simulink model "nonlinearized"  (R2020a)
settings: Solver=ode45  StartTime=0.0  StopTime=1000  FixedStep=0.01  MaxStep=0.05  RelTol=1e-3
undefined symbols (not defined in the file): auniversal, CLRolla20breakpoint1, CLRolla20breakpoint2, CLRolla20data, CLRollbreakpoint1, CLRollbreakpoint2, CLRolldata, CLRollPdata, CLRollr30breakpoint1, CLRollr30breakpoint2, CLRollr30data, CLRollRdata, CMbreakpoint1, CMbreakpoint2, CMdata, CMQdata, CNa20breakpoint1, CNa20breakpoint2, CNa20data, CNbreakpoint1, CNbreakpoint2, CNdata, CNPdata, CNr30breakpoint1, CNr30breakpoint2, CNr30data, CNRdata, CXbreakpoint1, CXbreakpoint2, CXdata, CXQdata, CYPdata, CYRdata, CZbreakpoint, CZdata, CZQdata, Tidlebreakpoint1, Tidlebreakpoint2, Tidledata, Tmaxbreakpoint1, Tmaxbreakpoint2, Tmaxdata, Tmilbreakpoint1, Tmilbreakpoint2, Tmildata, y
libraries: aerolibatmos2 x1
settings Model: Creator=WIN10  LastModifiedBy=WangLindong
settings DataIOCC: ReturnWorkspaceOutputs=off
settings DebuggingCC: InitInArrayFormatMsg=none  ArithmeticOperatorsInVariantConditions=warning
settings SFSimCC: SimUseLocalCustomCode=off  CustomCodeUndefinedFunction=UseInterfaceOnly
settings RTWCC: RTWUseLocalCustomCode=off
settings CodeAppCC: StateflowObjectComments=on
settings SimscapeCC: SimscapeNormalizeSystem=off

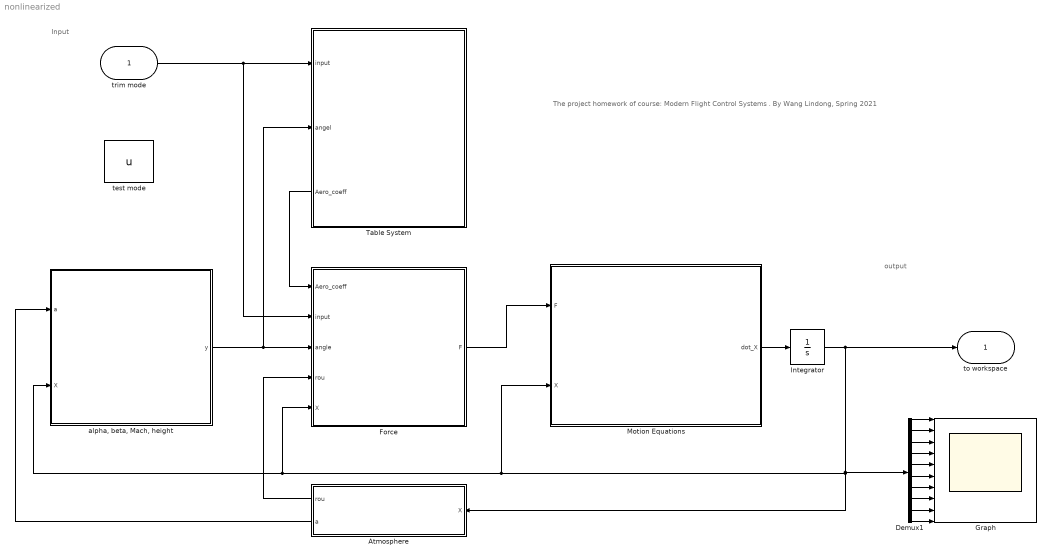
== system nonlinearized ==
  note: output
  note: Input
  note: The project homework of course: Modern Flight Control Systems . By Wang Lindong, Spring 2021
  trim mode : Inport
  Atmosphere : Subsystem
  Demux1 : Demux  Outputs=10
  Force : MATLAB Function  TreatAsAtomicUnit=on
  Graph : Scope  NumInputPorts=10
  Integrator : Integrator  InitialCondition=y
  Motion Equations : MATLAB Function  TreatAsAtomicUnit=on
  Table System : Subsystem
      settings: PortSchema="{\"entries\":[{\"content\":{\"sides\":[{\"content\":{\"connectorIds\":[\"In1\",\"In2\",\"Out1\"]},\"type\":\"ConnectorPlacement.EquallySpacedRectSide\",\"uuid\":\"a5097b1f-d505-459f-b2e6-571d27cac04d\"},{\"content\":{\"connectorIds\":[],\"side\":\"RIGHT\"},\"type\":\"ConnectorPlacement.EquallySpacedRectSide\",\"uuid\":\"94386472-c983-4c7e-a283-804fcfa61704\"},{\"content\":{\"connectorIds\":[],\"side\":\"TOP\"},\"type\":\"ConnectorPlacement.EquallySpacedRectSide\",\"uuid\":\"adeb2732-affa-4ea2-92b5-7f53d85af68a\"}]},\"type\":\"ConnectorPlacement.EquallySpacedConnector\",\"uuid\":\"5b9f7c15-7bde-4ddb-942d-45c343784d3d\"}],\"packageUris\":[\"http://schema.mathworks.com/mf0/Connector/19700101\"],\"version\":\"1.0\"}"
  "alpha, beta, Mach, height" : MATLAB Function  TreatAsAtomicUnit=on
  test mode : Constant  Value=u
  to workspace : Outport
  wires:
  Motion Equations/1(dot_X) -> Integrator/1
  Integrator/1 -> to workspace/1, Atmosphere/1(X), "alpha, beta, Mach, height"/2(X), Force/5(X), Motion Equations/2(X), Demux1/1
  Force/1(F) -> Motion Equations/1(F)
  Atmosphere/2(a) -> "alpha, beta, Mach, height"/1(a)
  Atmosphere/1(rou) -> Force/4(rou)
  trim mode/1 -> Force/2(input), Table System/1(input)
  Demux1/1 -> Graph/1
  Demux1/2 -> Graph/2
  Demux1/3 -> Graph/3
  Demux1/4 -> Graph/4
  Demux1/5 -> Graph/5
  Demux1/6 -> Graph/6
  Demux1/7 -> Graph/7
  Demux1/8 -> Graph/8
  Demux1/9 -> Graph/9
  Demux1/10 -> Graph/10
  Table System/1(Aero_coeff) -> Force/1(Aero_coeff)
  "alpha, beta, Mach, height"/1(y) -> Force/3(angle), Table System/2(angel)

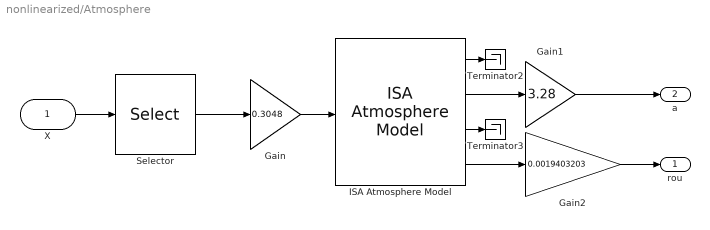
== system nonlinearized/Atmosphere ==
  X : Inport
  Gain : Gain  Gain=0.3048
  Gain1 : Gain  Gain=3.28
  Gain2 : Gain  Gain=0.0019403203
  ISA Atmosphere Model : aerolibatmos2/ISA Atmosphere Model  custom=off  g=9.80665  gamma=1.4  R=287.0531  L=0.0065  h_trop=11000  h_strat=20000  rho0=1.225  P0=101325  T0=288.15  h0=0
  Selector : Selector  InputPortWidth=10  IndexOptions=Index vector (dialog)  Indices=10  OutputSizes=1
  Terminator2 : Terminator
  Terminator3 : Terminator
  rou : Outport
  a : Outport  Port=2
  wires:
  X/1 -> Selector/1
  ISA Atmosphere Model/1 -> Terminator2/1
  ISA Atmosphere Model/4 -> Gain2/1
  Gain/1 -> ISA Atmosphere Model/1
  ISA Atmosphere Model/3 -> Terminator3/1
  ISA Atmosphere Model/2 -> Gain1/1
  Selector/1 -> Gain/1
  Gain1/1 -> a/1
  Gain2/1 -> rou/1

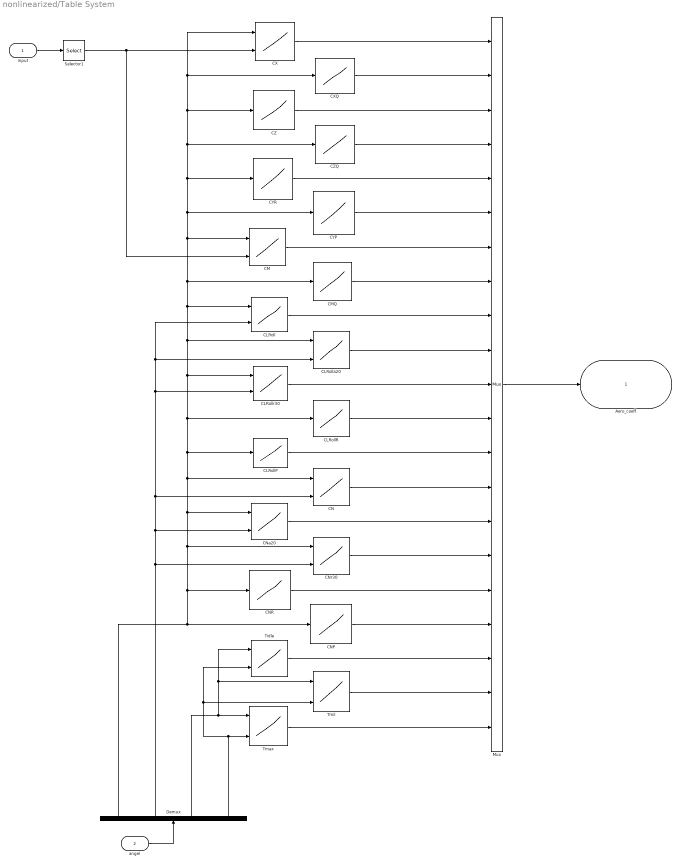
== system nonlinearized/Table System ==
  input : Inport
  angel : Inport  Port=2
  CLRoll : Lookup_n-D  BreakpointsForDimension1=CLRollbreakpoint1  BreakpointsForDimension2=CLRollbreakpoint2  Table=CLRolldata  InternalRulePriority=Speed  RndMeth=Simplest  InputSameDT=on
  CLRollP : Lookup_n-D  NumberOfTableDimensions=1  BreakpointsForDimension1=auniversal  Table=CLRollPdata  InternalRulePriority=Speed  RndMeth=Simplest  InputSameDT=on
  CLRollR : Lookup_n-D  NumberOfTableDimensions=1  BreakpointsForDimension1=auniversal  Table=CLRollRdata  InternalRulePriority=Speed  RndMeth=Simplest  InputSameDT=on
  CLRolla20 : Lookup_n-D  BreakpointsForDimension1=CLRolla20breakpoint1  BreakpointsForDimension2=CLRolla20breakpoint2  Table=CLRolla20data  InternalRulePriority=Speed  RndMeth=Simplest  InputSameDT=on
  CLRollr30 : Lookup_n-D  BreakpointsForDimension1=CLRollr30breakpoint1  BreakpointsForDimension2=CLRollr30breakpoint2  Table=CLRollr30data  InternalRulePriority=Speed  RndMeth=Simplest  InputSameDT=on
  CM : Lookup_n-D  BreakpointsForDimension1=CMbreakpoint1  BreakpointsForDimension2=CMbreakpoint2  Table=CMdata  InternalRulePriority=Speed  RndMeth=Simplest  InputSameDT=on
  CMQ : Lookup_n-D  NumberOfTableDimensions=1  BreakpointsForDimension1=auniversal  Table=CMQdata  InternalRulePriority=Speed  RndMeth=Simplest  InputSameDT=on
  CN : Lookup_n-D  BreakpointsForDimension1=CNbreakpoint1  BreakpointsForDimension2=CNbreakpoint2  Table=CNdata  InternalRulePriority=Speed  RndMeth=Simplest  InputSameDT=on
  CNP : Lookup_n-D  NumberOfTableDimensions=1  BreakpointsForDimension1=auniversal  Table=CNPdata  InternalRulePriority=Speed  RndMeth=Simplest  InputSameDT=on
  CNR : Lookup_n-D  NumberOfTableDimensions=1  BreakpointsForDimension1=auniversal  Table=CNRdata  InternalRulePriority=Speed  RndMeth=Simplest  InputSameDT=on
  CNa20 : Lookup_n-D  BreakpointsForDimension1=CNa20breakpoint1  BreakpointsForDimension2=CNa20breakpoint2  Table=CNa20data  InternalRulePriority=Speed  RndMeth=Simplest  InputSameDT=on
  CNr30 : Lookup_n-D  BreakpointsForDimension1=CNr30breakpoint1  BreakpointsForDimension2=CNr30breakpoint2  Table=CNr30data  InternalRulePriority=Speed  RndMeth=Simplest  InputSameDT=on
  CX : Lookup_n-D  BreakpointsForDimension1=CXbreakpoint1  BreakpointsForDimension2=CXbreakpoint2  Table=CXdata  InternalRulePriority=Speed  RndMeth=Simplest  InputSameDT=on
  CXQ : Lookup_n-D  NumberOfTableDimensions=1  BreakpointsForDimension1=auniversal  Table=CXQdata  InternalRulePriority=Speed  RndMeth=Simplest  InputSameDT=on
  CYP : Lookup_n-D  NumberOfTableDimensions=1  BreakpointsForDimension1=auniversal  Table=CYPdata  InternalRulePriority=Speed  RndMeth=Simplest  InputSameDT=on
  CYR : Lookup_n-D  NumberOfTableDimensions=1  BreakpointsForDimension1=auniversal  Table=CYRdata  InternalRulePriority=Speed  RndMeth=Simplest  InputSameDT=on
  CZ : Lookup_n-D  NumberOfTableDimensions=1  BreakpointsForDimension1=CZbreakpoint  Table=CZdata  InternalRulePriority=Speed  RndMeth=Simplest  InputSameDT=on
  CZQ : Lookup_n-D  NumberOfTableDimensions=1  BreakpointsForDimension1=auniversal  Table=CZQdata  InternalRulePriority=Speed  RndMeth=Simplest  InputSameDT=on
  Demux : Demux
  Mux : Mux  Inputs=21
  Selector1 : Selector  InputPortWidth=4  IndexOptions=Index vector (dialog)  Indices=1  OutputSizes=1
  Tidle : Lookup_n-D  BreakpointsForDimension1=Tidlebreakpoint1  BreakpointsForDimension2=Tidlebreakpoint2  Table=Tidledata  InternalRulePriority=Speed  RndMeth=Simplest  InputSameDT=on
  Tmax : Lookup_n-D  BreakpointsForDimension1=Tmaxbreakpoint1  BreakpointsForDimension2=Tmaxbreakpoint2  Table=Tmaxdata  InternalRulePriority=Speed  RndMeth=Simplest  InputSameDT=on
  Tmil : Lookup_n-D  BreakpointsForDimension1=Tmilbreakpoint1  BreakpointsForDimension2=Tmilbreakpoint2  Table=Tmildata  InternalRulePriority=Speed  RndMeth=Simplest  InputSameDT=on
  Aero_coeff : Outport
  wires:
  Tmax/1 -> Mux/21
  CN/1 -> Mux/14
  CXQ/1 -> Mux/2
  Tmil/1 -> Mux/20
  Demux/1 -> CNP/1, CNR/1, CNr30/1, CNa20/1, CN/1, CLRollP/1, CLRollR/1, CLRollr30/1, CLRolla20/1, CLRoll/1, CMQ/1, CM/1, CYP/1, CYR/1, CZQ/1, CZ/1, CXQ/1, CX/1
  CMQ/1 -> Mux/8
  Demux/4 -> Tmax/2, Tmil/2, Tidle/2
  Selector1/1 -> CX/2, CM/2
  Demux/3 -> Tidle/1, Tmil/1, Tmax/1
  CNP/1 -> Mux/18
  CNR/1 -> Mux/17
  CLRolla20/1 -> Mux/10
  CNr30/1 -> Mux/16
  CNa20/1 -> Mux/15
  CLRollR/1 -> Mux/12
  CLRollP/1 -> Mux/13
  CYP/1 -> Mux/6
  CZQ/1 -> Mux/4
  CM/1 -> Mux/7
  CLRoll/1 -> Mux/9
  CLRollr30/1 -> Mux/11
  Demux/2 -> CNr30/2, CNa20/2, CN/2, CLRollr30/2, CLRolla20/2, CLRoll/2
  CX/1 -> Mux/1
  CZ/1 -> Mux/3
  Tidle/1 -> Mux/19
  CYR/1 -> Mux/5
  Mux/1 -> Aero_coeff/1
  input/1 -> Selector1/1
  angel/1 -> Demux/1

== matlab function nonlinearized/Motion Equations ==
  data: F input; X input; dot_X output
function dot_X = fcn(F, X)
% X=[U V W P Q R fi theta xita h]'
g = 32.1520;
I = [9496,0,982;0,55814,0;982,0,63100];
m = 637.6;

t = zeros(10,1);
t(1) = -g*sin(X(8))+(F(1)+F(4))/m+(X(2)*X(6)-X(3)*X(5));
t(2) =  g*sin(X(7))*cos(X(8))+(F(2)+F(5))/m+(X(3)*X(4)-X(1)*X(6));
t(3) =  g*cos(X(7))*cos(X(8))+(F(3)+F(6))/m+(X(1)*X(5)-X(2)*X(4));
t(4) = -(I(3,3)*F(7) + I(3,3)*F(10) + I(3,1)*F(9) + I(3,1)*F(12) - I(3,1)^2*X(5)*X(6) - I(3,3)^2*X(5)*X(6) + I(1,1)*I(3,1)*X(4)*X(5) - I(3,1)*I(2,2)*X(4)*X(5) + I(3,1)*I(3,3)*X(4)*X(5) + I(2,2)*I(3,3)*X(5)*X(6))/(I(3,1)^2 - I(1,1)*I(3,3));
t(5) = (-X(4)*X(6)*(I(1,1)-I(3,3)) + (X(6)^2-X(4)^2)*I(3,1) + F(8) + F(11))/I(2,2);
t(6) = -(I(3,1)*F(7) + I(3,1)*F(10) + I(1,1)*F(9) + I(1,1)*F(12) + I(1,1)^2*X(4)*X(5) + I(3,1)^2*X(4)*X(5) - I(1,1)*I(2,2)*X(4)*X(5) - I(1,1)*I(3,1)*X(5)*X(6) + I(3,1)*I(2,2)*X(5)*X(6) - I(3,1)*I(3,3)*X(5)*X(6))/(I(3,1)^2 - I(1,1)*I(3,3));
t(7) = X(4) + sin(X(7))*tan(X(8))*X(5) + cos(X(7))*tan(X(8))*X(6);
t(8) = cos(X(7))*X(5)-sin(X(7))*X(6);
t(9) = sin(X(7))*sec(X(8))*X(5) + cos(X(7))*sec(X(8))*X(6);
t(10) = X(1)*sin(X(8))-X(2)*sin(X(7))*cos(X(8))-X(3)*cos(X(7))*cos(X(8));

X = t;
dot_X = X;

== matlab function nonlinearized/Force ==
  data: Aero_coeff input; input input; F output; angle input; rou input; X input
function F = fcn(Aero_coeff,input,angle,rou,X)
% F=[FAX,FAY,FAZ,FTX,FTY,FTZ,LA,MA,NA,LT,MT,NT]
% X=[U V W P Q R fi theta xita X Y h]
% input=sigma[e,a,r,T]

b = 30;
c = 11.32;
g = 32.1520;
S = 300;
xcg = 0.3;
xcgref = 0.35;
F = zeros(12,1);
V = sqrt(X(1)^2+X(2)^2+X(3)^2);
q = 0.5*(X(1)^2+X(3)^2)*rou;

CX = Aero_coeff(1);
CXQ = Aero_coeff(2);
CZ = Aero_coeff(3);
CZQ = Aero_coeff(4);
CYR = Aero_coeff(5);
CYP = Aero_coeff(6);
CM = Aero_coeff(7);
CMQ = Aero_coeff(8);
CLRoll = Aero_coeff(9);
CLRolla20 = Aero_coeff(10);
CLRollr30 = Aero_coeff(11);
CLRollR = Aero_coeff(12);
CLRollP = Aero_coeff(13);
CN = Aero_coeff(14);
CNa20 = Aero_coeff(15);
CNr30 = Aero_coeff(16);
CNR = Aero_coeff(17);
CNP = Aero_coeff(18);
Tidle = Aero_coeff(19);
Tmil = Aero_coeff(20);
Tmax = Aero_coeff(21);

beta = angle(2);

CXa = CX+c*X(5)/(2*V)*CXQ;
CZa = CZ*(1-(beta/57.3)^2)-0.19*input(1)/25+c*X(5)/(2*V)*CZQ;
CYa = (-0.02*beta+0.021*input(2)/20+0.86*input(3)/30)+b/(2*V)*(CYR*X(6)+CYP*X(4));
CMa = CM+c*X(5)/(2*V)*CMQ+CZa*(xcgref-xcg);
CLRolla = CLRoll+ CLRolla20*input(2)/20+ CLRollr30*input(3)/30 + b/(2*V)*(CLRollR*X(6)+CLRollP*X(4));
CNa = CN + CNa20*input(2)/20 + CNr30*input(3)/30 + b/(2*V)*(CNR*X(6)+CNP*X(4)) - CYa*(xcgref-xcg)*c/b;
F(1) = CXa*q*S;
F(2) = CYa*q*S;
F(3) = CZa*q*S;
F(7) = CLRolla*q*S*b;
F(8) = CMa*q*S*b;
F(9) = CNa*q*S*b;
if input(4)<0.77
    P = 64.94*input(4);
else
    P = 217.38*input(4)-117.38;
end

if P<50
    F(4) = Tidle+(Tmil-Tidle)*(P/50);
else
    F(4) = Tmil+(Tmax-Tmil)*(P-50)/50;
end
F = F;

== matlab function nonlinearized/alpha, beta, Mach, height ==
  data: a input; X input; y output
function y = fcn(a, X)
V = (X(1)^2+X(2)^2+X(3)^2)^0.5;%velocity
alpha = asin(X(3)/(X(1)^2+X(3)^2)^0.5)*180/pi;%beta
beta= asin(X(2)/V)*180/pi;%alpha
M = V/a;
h = X(10);
y = [alpha,beta,M,h];
